simulink model "HW4_model"  (R2021b)
settings: Solver=ode4  StartTime=0.0  StopTime=5  FixedStep=h  RelTol=1e-3
values from neighbouring files (symbols this model uses):
  aug_sim_states = X(1:3,:)    [HW4.m]
  nonaug_sim_states = X(1:3,:)    [HW4.m]
  time = 0:h:5    [HW4.m]
libraries: vrlib x2
settings Model: Creator=17165  LastModifiedBy=17165

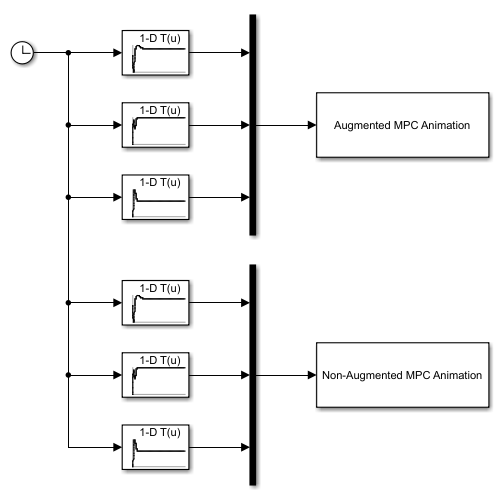
[thumbnail: Simulink's stored preview of the top-level diagram]
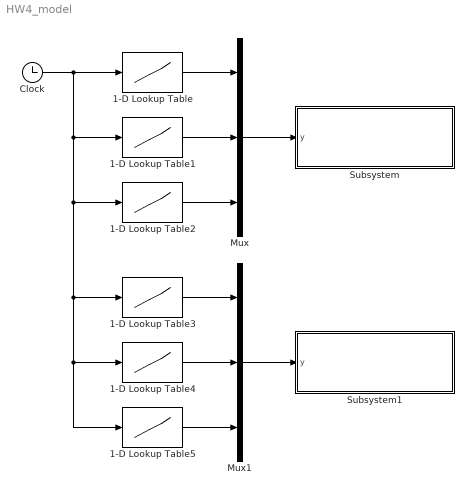
== system HW4_model ==
  1-D Lookup Table : Lookup_n-D  NumberOfTableDimensions=1  BreakpointsForDimension1=time  Table=aug_sim_states(1,:)  InternalRulePriority=Speed  RndMeth=Simplest  InputSameDT=on
  1-D Lookup Table1 : Lookup_n-D  NumberOfTableDimensions=1  BreakpointsForDimension1=time  Table=aug_sim_states(2,:)  InternalRulePriority=Speed  RndMeth=Simplest  InputSameDT=on
  1-D Lookup Table2 : Lookup_n-D  NumberOfTableDimensions=1  BreakpointsForDimension1=time  Table=aug_sim_states(3,:)  InternalRulePriority=Speed  RndMeth=Simplest  InputSameDT=on
  1-D Lookup Table3 : Lookup_n-D  NumberOfTableDimensions=1  BreakpointsForDimension1=time  Table=nonaug_sim_states(1,:)  InternalRulePriority=Speed  RndMeth=Simplest  InputSameDT=on
  1-D Lookup Table4 : Lookup_n-D  NumberOfTableDimensions=1  BreakpointsForDimension1=time  Table=nonaug_sim_states(2,:)  InternalRulePriority=Speed  RndMeth=Simplest  InputSameDT=on
  1-D Lookup Table5 : Lookup_n-D  NumberOfTableDimensions=1  BreakpointsForDimension1=time  Table=nonaug_sim_states(3,:)  InternalRulePriority=Speed  RndMeth=Simplest  InputSameDT=on
  Clock : Clock
  Mux : Mux  Inputs=3
  Mux1 : Mux  Inputs=3
  Subsystem : Subsystem
      mask Display: disp('Augmented MPC Animation')
  Subsystem1 : Subsystem
      mask Display: disp('Non-Augmented MPC Animation')
  wires:
  1-D Lookup Table1/1 -> Mux/2
  1-D Lookup Table/1 -> Mux/1
  1-D Lookup Table2/1 -> Mux/3
  Mux/1 -> Subsystem/1(y)
  1-D Lookup Table5/1 -> Mux1/3
  Clock/1 -> 1-D Lookup Table5/1, 1-D Lookup Table4/1, 1-D Lookup Table3/1, 1-D Lookup Table2/1, 1-D Lookup Table1/1, 1-D Lookup Table/1
  1-D Lookup Table3/1 -> Mux1/1
  1-D Lookup Table4/1 -> Mux1/2
  Mux1/1 -> Subsystem1/1(y)

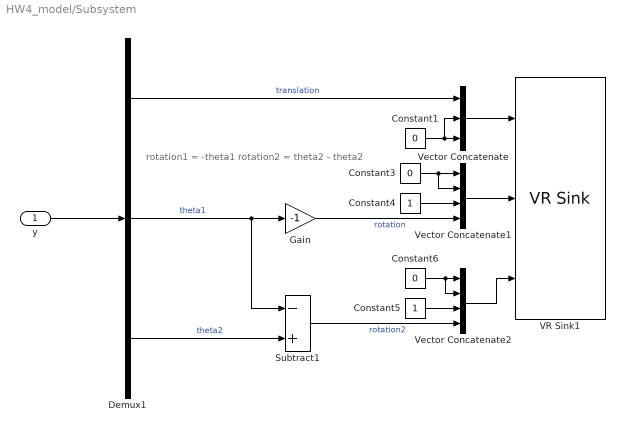
== system HW4_model/Subsystem ==
  note: rotation1 = -theta1
      | rotation2 = theta2 - theta2
  y : Inport
  Constant1 : Constant  Value=0
  Constant3 : Constant  Value=0
  Constant4 : Constant
  Constant5 : Constant
  Constant6 : Constant  Value=0
  Demux1 : Demux  Outputs=3
  Gain : Gain  Gain=-1
  Subtract1 : Sum  Inputs=-+
  VR Sink1 : vrlib/VR Sink  InstantiateOnLoad=on  SampleTime=-1  ViewEnable=on  RemoteChange=off  RemoteView=off  FieldsWritten=Cart.translation.3.1.1.double#Rotation1.rotation.4.1.1.double#Rotation2.rotation.4.1.1.double  WorldFileName=DIPC.x3d  AutoView=off  VideoDimensions=[]  AllowVariableSize=off  FigureProperties="{'Position', 'Name', 'Viewpoint', 'CameraBound', 'CameraDirection', 'CameraPosition', 'CameraUpVector', 'ZoomFactor', 'Antialiasing', 'Headlight', 'Lighting', 'NavPanel', 'Sound', 'StatusBar', 'Stereo3D', 'Stereo3DCameraOffset', 'Stereo3DHIT', 'ToolBar', 'Textures', 'Transparency', 'Triad', 'Wireframe', 'NavZones', 'NavMode', 'NavSpeed', 'CaptureFileFormat', 'CaptureFileName', 'Record2DCompressMethod', 'Record2DCompressQuality', 'Record2D', 'Record2DFileName', 'Record2DFPS'; [5.0000000000000000e+00   9.2000000000000000e+01   5.7600000000000000e+02   3.5000000000000000e+02], '', '_untitled_1', 'on', [0.0000000000000000e+00   0.0000000000000000e+00  -1.0000000000000000e+00], [0.0000000000000000e+00   0.0000000000000000e+00   0.0000000000000000e+00], [0.0000000000000000e+00   1.0000000000000000e+00   0.0000000000000000e+00], [1.0000000000000000e+00], 'on', 'on', 'on', 'halfbar', 'on', 'on', 'off', [1.0000000149011612e-01], [0.0000000000000000e+00], 'on', 'on', 'on', 'none', 'off', 'off', 'fly', 'normal', 'tif', '%f_anim_%n.tif', 'auto', [7.5000000000000000e+01], 'on', 'AugmentedSystem.avi', 'auto'}"
  Vector Concatenate : Concatenate  NumInputs=3
  Vector Concatenate1 : Concatenate  NumInputs=4
  Vector Concatenate2 : Concatenate  NumInputs=4
  wires:
  Constant3/1 -> Vector Concatenate1/2, Vector Concatenate1/1
  Gain/1 -> Vector Concatenate1/4  "rotation"
  Constant4/1 -> Vector Concatenate1/3
  Constant1/1 -> Vector Concatenate/2, Vector Concatenate/3
  Demux1/2 -> Subtract1/1, Gain/1  "theta1"
  Demux1/3 -> Subtract1/2  "theta2"
  y/1 -> Demux1/1
  Subtract1/1 -> Vector Concatenate2/4  "rotation2"
  Vector Concatenate1/1 -> VR Sink1/2
  Vector Concatenate2/1 -> VR Sink1/3
  Vector Concatenate/1 -> VR Sink1/1
  Demux1/1 -> Vector Concatenate/1  "translation"
  Constant5/1 -> Vector Concatenate2/3
  Constant6/1 -> Vector Concatenate2/2, Vector Concatenate2/1

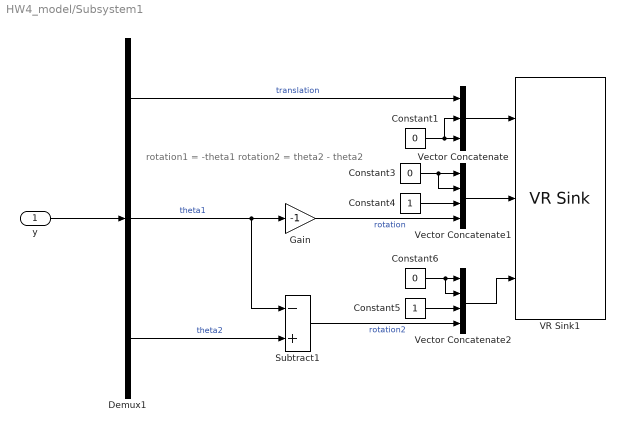
== system HW4_model/Subsystem1 ==
  note: rotation1 = -theta1
      | rotation2 = theta2 - theta2
  y : Inport
  Constant1 : Constant  Value=0
  Constant3 : Constant  Value=0
  Constant4 : Constant
  Constant5 : Constant
  Constant6 : Constant  Value=0
  Demux1 : Demux  Outputs=3
  Gain : Gain  Gain=-1
  Subtract1 : Sum  Inputs=-+
  VR Sink1 : vrlib/VR Sink  InstantiateOnLoad=on  SampleTime=-1  ViewEnable=on  RemoteChange=off  RemoteView=off  FieldsWritten=Cart.translation.3.1.1.double#Rotation1.rotation.4.1.1.double#Rotation2.rotation.4.1.1.double  WorldFileName=DIPC.x3d  AutoView=off  VideoDimensions=[]  AllowVariableSize=off  FigureProperties="{'Position', 'Name', 'Viewpoint', 'CameraBound', 'CameraDirection', 'CameraPosition', 'CameraUpVector', 'ZoomFactor', 'Antialiasing', 'Headlight', 'Lighting', 'NavPanel', 'Sound', 'StatusBar', 'Stereo3D', 'Stereo3DCameraOffset', 'Stereo3DHIT', 'ToolBar', 'Textures', 'Transparency', 'Triad', 'Wireframe', 'NavZones', 'NavMode', 'NavSpeed', 'CaptureFileFormat', 'CaptureFileName', 'Record2DCompressMethod', 'Record2DCompressQuality', 'Record2D', 'Record2DFileName', 'Record2DFPS'; [5.0000000000000000e+00   9.2000000000000000e+01   5.7600000000000000e+02   3.5000000000000000e+02], '', '_untitled_1', 'on', [0.0000000000000000e+00   0.0000000000000000e+00  -1.0000000000000000e+00], [0.0000000000000000e+00   0.0000000000000000e+00   0.0000000000000000e+00], [0.0000000000000000e+00   1.0000000000000000e+00   0.0000000000000000e+00], [1.0000000000000000e+00], 'on', 'on', 'on', 'halfbar', 'on', 'on', 'off', [1.0000000149011612e-01], [0.0000000000000000e+00], 'on', 'on', 'on', 'none', 'off', 'off', 'fly', 'normal', 'tif', '%f_anim_%n.tif', 'auto', [7.5000000000000000e+01], 'on', 'NonAugmentedSystem.avi', 'auto'}"
  Vector Concatenate : Concatenate  NumInputs=3
  Vector Concatenate1 : Concatenate  NumInputs=4
  Vector Concatenate2 : Concatenate  NumInputs=4
  wires:
  Constant3/1 -> Vector Concatenate1/2, Vector Concatenate1/1
  Gain/1 -> Vector Concatenate1/4  "rotation"
  Constant4/1 -> Vector Concatenate1/3
  Constant1/1 -> Vector Concatenate/2, Vector Concatenate/3
  Demux1/2 -> Subtract1/1, Gain/1  "theta1"
  Demux1/3 -> Subtract1/2  "theta2"
  y/1 -> Demux1/1
  Subtract1/1 -> Vector Concatenate2/4  "rotation2"
  Vector Concatenate1/1 -> VR Sink1/2
  Vector Concatenate2/1 -> VR Sink1/3
  Vector Concatenate/1 -> VR Sink1/1
  Demux1/1 -> Vector Concatenate/1  "translation"
  Constant5/1 -> Vector Concatenate2/3
  Constant6/1 -> Vector Concatenate2/2, Vector Concatenate2/1
